simulink model "CaseStudyI_9_Bus"  (R2020a)
settings: Solver=FixedStepAuto  StartTime=0.0  StopTime=Tend  FixedStep=T_s_power  MaxStep=5.0E-5  RelTol=1e-3
values from neighbouring files (symbols this model uses):
  B_s46 = b_s46*Cb    (= 9.5071761847e-07)    [Data_CaseStudyI.m]    (also in Data_CaseStudyII.m; Data_InitialSystem.m)
  B_s54 = b_s54*Cb    (= 1.05902722057e-06)    [Data_CaseStudyI.m]    (also in Data_CaseStudyII.m; Data_InitialSystem.m)
  B_s69 = b_s69*Cb    (= 2.15415764185e-06)    [Data_CaseStudyI.m]    (also in Data_CaseStudyII.m; Data_InitialSystem.m)
  B_s75 = b_s75*Cb    (= 1.84126323577e-06)    [Data_CaseStudyI.m]    (also in Data_CaseStudyII.m; Data_InitialSystem.m)
  B_s87 = b_s87*Cb    (= 8.96562817417e-07)    [Data_CaseStudyI.m]    (also in Data_CaseStudyII.m; Data_InitialSystem.m)
  B_s98 = b_s98*Cb    (= 1.25759482443e-06)    [Data_CaseStudyI.m]    (also in Data_CaseStudyII.m; Data_InitialSystem.m)
  C_dc_DVPP_1_2 = 0.008*(n_DVPP_1_2)    (= 0.8)    [Data_CaseStudyI.m]    (also in Data_CaseStudyII.m)
  C_dc_DVPP_1_3 = 0.008*(n_DVPP_1_3)    (= 0.4)    [Data_CaseStudyI.m]    (also in Data_CaseStudyII.m)
  fb = 50    [Data_CaseStudyI.m]    (also in Data_CaseStudyII.m; Data_InitialSystem.m)
  HGov_dyn = HGov_delay*H_tr_droop    [Data_CaseStudyI.m]    (also in Data_CaseStudyII.m; Data_InitialSystem.m)
  HTurb_tot = H_water_way    [Data_CaseStudyI.m]    (also in Data_CaseStudyII.m; Data_InitialSystem.m)
  I_m_DVPP_1_2 = 2/3*Sb_DVPP_1_2/V_m_DVPP_1_2    [Data_CaseStudyI.m]    (also in Data_CaseStudyII.m)
  I_m_DVPP_1_3 = 2/3*Sb_DVPP_1_3/V_m_DVPP_1_3    [Data_CaseStudyI.m]    (also in Data_CaseStudyII.m)
  i_star_max = 1.3    [Data_CaseStudyI.m]    (also in Data_CaseStudyII.m)
  iabc_DVPP_1_2_0 = T0*idq0_DVPP_1_2    [Data_CaseStudyI.m]    (also in Data_CaseStudyII.m)
  iabc_DVPP_1_3_0 = T0*idq0_DVPP_1_3    [Data_CaseStudyI.m]    (also in Data_CaseStudyII.m)
  K2_DVPP_1 = [-0.0221795494247 -1.60799665656 0.160449825826 -2.94803557381 -11.8081988371 -9.75170960256 0.00463021906909 -49.1667298155]    [ControlGains_DVPP1.mat]
  K3_DVPP_1 = [-0.0591512752956 -1.61493903379 -27.2946107927 -16.2119211358 -14.3657419818 2.05688388773 -2.27328406162 0.146700393037 -150.920793597]    [ControlGains_DVPP1.mat]
  k_dc_DVPP_1_2 = eta_DVPP_1_2/(Vdc_n_DVPP_1_2*m_p_DVPP_1_2)    [Data_CaseStudyI.m]    (also in Data_CaseStudyII.m)
  k_dc_DVPP_1_3 = eta_DVPP_1_3/(Vdc_n_DVPP_1_3*m_p_DVPP_1_3)    [Data_CaseStudyI.m]    (also in Data_CaseStudyII.m)
  ki_i_pu = 1.19    [Data_CaseStudyI.m]    (also in Data_CaseStudyII.m)
  ki_pll = 1700    [Data_CaseStudyI.m]    (also in Data_CaseStudyII.m)
  ki_q_pu = 0.005    [Data_CaseStudyI.m]    (also in Data_CaseStudyII.m)
  kp_i_pu = 0.73    [Data_CaseStudyI.m]    (also in Data_CaseStudyII.m)
  kp_pll = 150    [Data_CaseStudyI.m]    (also in Data_CaseStudyII.m)
  kp_q_pu = 0.05    [Data_CaseStudyI.m]    (also in Data_CaseStudyII.m)
  L1_DVPP_1_2_pu = 0.0186/m_DVPP_1_2    (= 0.000372)    [Data_CaseStudyI.m]    (also in Data_CaseStudyII.m)
  L1_DVPP_1_3_pu = 0.0186/m_DVPP_1_3    (= 0.000744)    [Data_CaseStudyI.m]    (also in Data_CaseStudyII.m)
  l1_MVHV1 = 0    [Data_CaseStudyI.m]    (also in Data_CaseStudyII.m; Data_InitialSystem.m)
  l1_MVHV2 = 0    [Data_CaseStudyI.m]    (also in Data_CaseStudyII.m; Data_InitialSystem.m)
  l1_MVHV3 = 0    [Data_CaseStudyI.m]    (also in Data_CaseStudyII.m; Data_InitialSystem.m)
  L2_DVPP_1_2_pu = L1_DVPP_1_2_pu    (= 0.000372)    [Data_CaseStudyI.m]    (also in Data_CaseStudyII.m)
  L2_DVPP_1_3_pu = L1_DVPP_1_3_pu    (= 0.000744)    [Data_CaseStudyI.m]    (also in Data_CaseStudyII.m)
  l2_MVHV1 = l_s14    (= 0.0576)    [Data_CaseStudyI.m]    (also in Data_CaseStudyII.m; Data_InitialSystem.m)
  l2_MVHV2 = l_s72    (= 0.0625)    [Data_CaseStudyI.m]    (also in Data_CaseStudyII.m; Data_InitialSystem.m)
  l2_MVHV3 = l_s39    (= 0.0586)    [Data_CaseStudyI.m]    (also in Data_CaseStudyII.m; Data_InitialSystem.m)
  l_f_DVPP_1_2 = L_f_DVPP_1_2*w_b/Zb_DVPP_1_2    [Data_CaseStudyI.m]    (also in Data_CaseStudyII.m)
  L_f_DVPP_1_2 = (1/(n_DVPP_1_2))*600*10^-6    (= 6e-06)    [Data_CaseStudyI.m]    (also in Data_CaseStudyII.m)
  l_f_DVPP_1_3 = L_f_DVPP_1_3*w_b/Zb_DVPP_1_3    [Data_CaseStudyI.m]    (also in Data_CaseStudyII.m)
  L_f_DVPP_1_3 = (1/(n_DVPP_1_3))*600*10^-6    (= 1.2e-05)    [Data_CaseStudyI.m]    (also in Data_CaseStudyII.m)
  L_s46 = l_s46*Lb    (= 0.154915055408)    [Data_CaseStudyI.m]    (also in Data_CaseStudyII.m; Data_InitialSystem.m)
  L_s54 = l_s54*Lb    (= 0.143128040323)    [Data_CaseStudyI.m]    (also in Data_CaseStudyII.m; Data_InitialSystem.m)
  L_s69 = l_s69*Lb    (= 0.286256080645)    [Data_CaseStudyI.m]    (also in Data_CaseStudyII.m; Data_InitialSystem.m)
  L_s75 = l_s75*Lb    (= 0.271101346964)    [Data_CaseStudyI.m]    (also in Data_CaseStudyII.m; Data_InitialSystem.m)
  L_s87 = l_s87*Lb    (= 0.12123786945)    [Data_CaseStudyI.m]    (also in Data_CaseStudyII.m; Data_InitialSystem.m)
  L_s98 = l_s98*Lb    (= 0.16973301723)    [Data_CaseStudyI.m]    (also in Data_CaseStudyII.m; Data_InitialSystem.m)
  P_L = pL*Sb    (= 300000000)    [Data_CaseStudyI.m]    (also in Data_CaseStudyII.m; Data_InitialSystem.m)
  p_set_bus1 = P_set_bus1/SbSG1    (= 0.731707317073)    [Data_CaseStudyI.m]    (also in Data_CaseStudyII.m; Data_InitialSystem.m)
  p_set_bus2 = P_set_bus2/SbSG2    (= 0.756707317073)    [Data_CaseStudyI.m]    (also in Data_CaseStudyII.m; Data_InitialSystem.m)
  p_set_bus3 = P_set_bus3/SbSG3    (= 0.731707317073)    [Data_CaseStudyI.m]    (also in Data_CaseStudyII.m; Data_InitialSystem.m)
  pset_DVPP_1_1 = P_set_bus1/SbSG1    (= 0.731707317073)    [Data_CaseStudyI.m]    (also in Data_CaseStudyII.m)
  pset_DVPP_1_2 = 0    [Data_CaseStudyI.m]    (also in Data_CaseStudyII.m)
  pset_DVPP_1_3 = 0    [Data_CaseStudyI.m]    (also in Data_CaseStudyII.m)
  Q_L = qL*Sb    (= 82500000)    [Data_CaseStudyI.m]    (also in Data_CaseStudyII.m; Data_InitialSystem.m)
  qset_DVPP_1_2 = 0    [Data_CaseStudyI.m]    (also in Data_CaseStudyII.m)
  qset_DVPP_1_3 = 0    [Data_CaseStudyI.m]    (also in Data_CaseStudyII.m)
  R1_DVPP_1_2_pu = 0.00734/m_DVPP_1_2    (= 0.0001468)    [Data_CaseStudyI.m]    (also in Data_CaseStudyII.m)
  R1_DVPP_1_3_pu = 0.00734/m_DVPP_1_3    (= 0.0002936)    [Data_CaseStudyI.m]    (also in Data_CaseStudyII.m)
  r1_MVHV1 = 1e-6    (= 1e-06)    [Data_CaseStudyI.m]    (also in Data_CaseStudyII.m; Data_InitialSystem.m)
  r1_MVHV2 = 1e-6    (= 1e-06)    [Data_CaseStudyI.m]    (also in Data_CaseStudyII.m; Data_InitialSystem.m)
  r1_MVHV3 = 1e-6    (= 1e-06)    [Data_CaseStudyI.m]    (also in Data_CaseStudyII.m; Data_InitialSystem.m)
  R2_DVPP_1_2_pu = R1_DVPP_1_2_pu    (= 0.0001468)    [Data_CaseStudyI.m]    (also in Data_CaseStudyII.m)
  R2_DVPP_1_3_pu = R1_DVPP_1_3_pu    (= 0.0002936)    [Data_CaseStudyI.m]    (also in Data_CaseStudyII.m)
  r2_MVHV1 = 1e-6    (= 1e-06)    [Data_CaseStudyI.m]    (also in Data_CaseStudyII.m; Data_InitialSystem.m)
  r2_MVHV2 = 1e-6    (= 1e-06)    [Data_CaseStudyI.m]    (also in Data_CaseStudyII.m; Data_InitialSystem.m)
  r2_MVHV3 = 1e-6    (= 1e-06)    [Data_CaseStudyI.m]    (also in Data_CaseStudyII.m; Data_InitialSystem.m)
  R_dc_DVPP_1_2 = (Vdc_n_DVPP_1_2/(0.05*(Sb_DVPP_1_2)/Vdc_n_DVPP_1_2))    [Data_CaseStudyI.m]    (also in Data_CaseStudyII.m)
  R_dc_DVPP_1_3 = (Vdc_n_DVPP_1_3/(0.05*(Sb_DVPP_1_3)/Vdc_n_DVPP_1_3))    [Data_CaseStudyI.m]    (also in Data_CaseStudyII.m)
  r_f_DVPP_1_2 = R_f_DVPP_1_2/Zb_DVPP_1_2    [Data_CaseStudyI.m]    (also in Data_CaseStudyII.m)
  R_f_DVPP_1_2 = 0.02/n_DVPP_1_2    (= 0.0002)    [Data_CaseStudyI.m]    (also in Data_CaseStudyII.m)
  r_f_DVPP_1_3 = R_f_DVPP_1_3/Zb_DVPP_1_3    [Data_CaseStudyI.m]    (also in Data_CaseStudyII.m)
  R_f_DVPP_1_3 = 0.02/n_DVPP_1_3    (= 0.0004)    [Data_CaseStudyI.m]    (also in Data_CaseStudyII.m)
  R_s46 = r_s46*Zb    (= 8.993)    [Data_CaseStudyI.m]    (also in Data_CaseStudyII.m; Data_InitialSystem.m)
  R_s54 = r_s54*Zb    (= 5.29)    [Data_CaseStudyI.m]    (also in Data_CaseStudyII.m; Data_InitialSystem.m)
  R_s69 = r_s69*Zb    (= 20.631)    [Data_CaseStudyI.m]    (also in Data_CaseStudyII.m; Data_InitialSystem.m)
  R_s75 = r_s75*Zb    (= 16.928)    [Data_CaseStudyI.m]    (also in Data_CaseStudyII.m; Data_InitialSystem.m)
  R_s87 = r_s87*Zb    (= 4.4965)    [Data_CaseStudyI.m]    (also in Data_CaseStudyII.m; Data_InitialSystem.m)
  R_s98 = r_s98*Zb    (= 6.2951)    [Data_CaseStudyI.m]    (also in Data_CaseStudyII.m; Data_InitialSystem.m)
  ReferenceSS2_DVPP_1 = ss(M2T_des_DVPP_1,'minimal')    [Data_CaseStudyI.m]    (also in Data_CaseStudyII.m)
  ReferenceSS3_DVPP_1 = ss(M3T_des_DVPP_1,'minimal')    [Data_CaseStudyI.m]    (also in Data_CaseStudyII.m)
  Rg = 0.03    [Data_CaseStudyI.m]    (also in Data_CaseStudyII.m; Data_InitialSystem.m)
  Sb = 100*10^6    (= 100000000)    [Data_CaseStudyI.m]    (also in Data_CaseStudyII.m; Data_InitialSystem.m)
  Sb_DVPP_1_2 = r_b1*100*10^6*cDVPP_1_2    (= 50000000)    [Data_CaseStudyI.m]    (also in Data_CaseStudyII.m)
  Sb_DVPP_1_3 = r_b1*100*10^6*cDVPP_1_3    (= 25000000)    [Data_CaseStudyI.m]    (also in Data_CaseStudyII.m)
  SbSG1 = r_b1*100*10^6    (= 250000000)    [Data_CaseStudyI.m]    (also in Data_CaseStudyII.m; Data_InitialSystem.m)
  SbSG2 = r_b2*100*10^6    (= 96000000)    [Data_CaseStudyI.m]    (also in Data_CaseStudyII.m; Data_InitialSystem.m)
  SbSG3 = r_b3*100*10^6    (= 64000000)    [Data_CaseStudyI.m]    (also in Data_CaseStudyII.m; Data_InitialSystem.m)
  SGov_dyn = tf([1],[Tg 1])    [Data_CaseStudyI.m]    (also in Data_CaseStudyII.m; Data_InitialSystem.m)
  St_MVHV1 = Sb    (= 100000000)    [Data_CaseStudyI.m]    (also in Data_CaseStudyII.m; Data_InitialSystem.m)
  St_MVHV2 = Sb    (= 100000000)    [Data_CaseStudyI.m]    (also in Data_CaseStudyII.m; Data_InitialSystem.m)
  St_MVHV3 = Sb    (= 100000000)    [Data_CaseStudyI.m]    (also in Data_CaseStudyII.m; Data_InitialSystem.m)
  St_MVLV_DVPP_1_2 = St*m_DVPP_1_2    (= 50000000)    [Data_CaseStudyI.m]    (also in Data_CaseStudyII.m)
  St_MVLV_DVPP_1_3 = St*m_DVPP_1_3    (= 25000000)    [Data_CaseStudyI.m]    (also in Data_CaseStudyII.m)
  STurb_reheat = STurb_ch*STurb_rh    [Data_CaseStudyI.m]    (also in Data_CaseStudyII.m; Data_InitialSystem.m)
  T_load_b3 = 2010    [Data_CaseStudyI.m]    (also in Data_CaseStudyII.m = 1010)
  T_load_b6 = 1010    [Data_CaseStudyI.m]    (also in Data_InitialSystem.m)
  T_s_power = 1e-4    (= 0.0001)    [Data_CaseStudyI.m]    (also in Data_CaseStudyII.m; Data_InitialSystem.m)
  tau_dc_DVPP_1_2 = 0.2    [Data_CaseStudyI.m]    (also in Data_CaseStudyII.m)
  tau_dc_DVPP_1_3 = 0.01    [Data_CaseStudyI.m]    (also in Data_CaseStudyII.m)
  V_m_DVPP_1_2 = VbLV_DVPP_1_2*sqrt(2/3)    [Data_CaseStudyI.m]    (also in Data_CaseStudyII.m)
  V_m_DVPP_1_3 = VbLV_DVPP_1_3*sqrt(2/3)    [Data_CaseStudyI.m]    (also in Data_CaseStudyII.m)
  vabc_DVPP_1_2_0_pu = T0*vdq0_DVPP_1_2_0/V_m_DVPP_1_2    [Data_CaseStudyI.m]    (also in Data_CaseStudyII.m)
  vabc_DVPP_1_3_0_pu = T0*vdq0_DVPP_1_3_0/V_m_DVPP_1_3    [Data_CaseStudyI.m]    (also in Data_CaseStudyII.m)
  VbHV = 230*10^3    (= 230000)    [Data_CaseStudyI.m]    (also in Data_CaseStudyII.m; Data_InitialSystem.m)
  VbLV_DVPP_1_2 = 10^3    (= 1000)    [Data_CaseStudyI.m]    (also in Data_CaseStudyII.m)
  VbLV_DVPP_1_3 = 10^3    (= 1000)    [Data_CaseStudyI.m]    (also in Data_CaseStudyII.m)
  VbMV1 = 16.5*10^3    (= 16500)    [Data_CaseStudyI.m]    (also in Data_CaseStudyII.m; Data_InitialSystem.m)
  VbMV2 = 18.0*10^3    (= 18000)    [Data_CaseStudyI.m]    (also in Data_CaseStudyII.m; Data_InitialSystem.m)
  VbMV3 = 13.8*10^3    (= 13800)    [Data_CaseStudyI.m]    (also in Data_CaseStudyII.m; Data_InitialSystem.m)
  vd0_DVPP_1_2_pu = vd0_DVPP_1_2/V_m_DVPP_1_2    [Data_CaseStudyI.m]    (also in Data_CaseStudyII.m)
  vd0_DVPP_1_3_pu = vd0_DVPP_1_3/V_m_DVPP_1_3    [Data_CaseStudyI.m]    (also in Data_CaseStudyII.m)
  Vdc_n_DVPP_1_2 = 3*V_m_DVPP_1_2    [Data_CaseStudyI.m]    (also in Data_CaseStudyII.m)
  Vdc_n_DVPP_1_3 = 3*V_m_DVPP_1_3    [Data_CaseStudyI.m]    (also in Data_CaseStudyII.m)
  w_b = fb*2*pi    (= 314.159265359)    [Data_CaseStudyI.m]    (also in Data_CaseStudyII.m; Data_InitialSystem.m)
  xid0_DVPP_1_2_pu = 0    [Data_CaseStudyI.m]    (also in Data_CaseStudyII.m)
  xid0_DVPP_1_3_pu = 0    [Data_CaseStudyI.m]    (also in Data_CaseStudyII.m)
  xiq0_DVPP_1_2_pu = 0    [Data_CaseStudyI.m]    (also in Data_CaseStudyII.m)
  xiq0_DVPP_1_3_pu = 0    [Data_CaseStudyI.m]    (also in Data_CaseStudyII.m)
  xpll0_pu = w_b/(ki_pll)    (= 0.184799567858)    [Data_CaseStudyI.m]    (also in Data_CaseStudyII.m)
  xq0_DVPP_1_2_pu = xq0_DVPP_1_2/I_m_DVPP_1_2    [Data_CaseStudyI.m]    (also in Data_CaseStudyII.m)
  ... (+1 more)
undefined symbols (not defined in the file or in its folder): A, B, C, Continuous, Dd, Efd0, gcbh, i_dc, Ka, Kf, p2set, SbSM2, sps_rtmsupport, spsST1AModel, Ta, Tb, Tb1, Tc, Tc1, Tf, VA0, VAmax, VAmin, VImax, VImin, VRmax, VRmin
libraries: powerlib x73, powerlib_meascontrol x16, cstblocks x11, sps_avr x2, simulink_extras x1, simulink x1
(part 2 of 3)

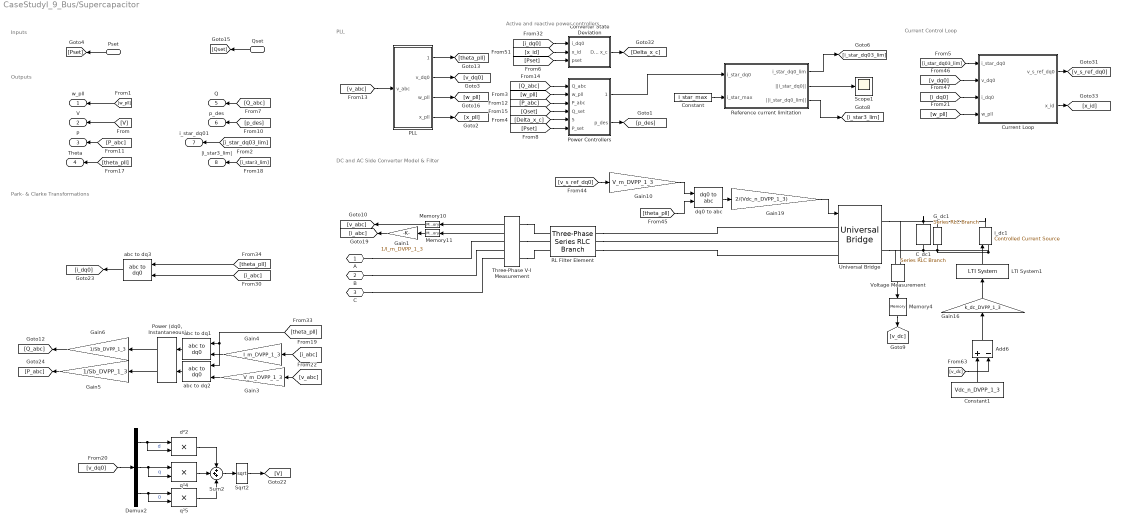
== system CaseStudyI_9_Bus/Supercapacitor ==
  note: Inputs
  note: Active and reactive power controllers
  note: PLL
  note: Outputs
  note: Current Control Loop
  note: Park- & Clarke Transformations
  note: DC and AC Side Converter Model & Filter
  Qset : Inport
  Pset : Inport  Port=2
  Add6 : Sum  Inputs=+-
  C_dc1 : powerlib/Elements/Series RLC Branch  LConnTagsString=__new0  RConnTagsString=__new0  BranchType=C  Resistance=1  Inductance=1e-3  SetiL0=off  InitialCurrent=0  Capacitance=C_dc_DVPP_1_3  Setx0=off  InitialVoltage=Vdc_n  Measurements=None
  Constant : Constant  Value=i_star_max
  Constant1 : Constant  Value=Vdc_n_DVPP_1_3
  Converter State Deviation : Subsystem
  Current Loop : Subsystem  AncestorBlock=Library/Grid-Forming Converter Controlled by Droop Control /Current Loop
  Demux2 : Demux  Outputs=3
  G_dc1 : powerlib/Elements/Series RLC Branch  LConnTagsString=__new0  RConnTagsString=__new0  BranchType=R  Resistance=R_dc_DVPP_1_3  Inductance=1e-3  SetiL0=off  InitialCurrent=0  Capacitance=1e-6  Setx0=off  InitialVoltage=0  Measurements=None
  Gain1 : Gain  Gain=1/I_m_DVPP_1_3
  Gain10 : Gain  Gain=V_m_DVPP_1_3
  Gain16 : Gain  Gain=k_dc_DVPP_1_3
  Gain19 : Gain  Gain=2/(Vdc_n_DVPP_1_3)
  Gain3 : Gain  Gain=V_m_DVPP_1_3
  Gain4 : Gain  Gain=I_m_DVPP_1_3
  Gain5 : Gain  Gain=1/Sb_DVPP_1_3
  Gain6 : Gain  Gain=1/Sb_DVPP_1_3
  LTI System1 : cstblocks/LTI System  sys=tf(1,[tau_dc_DVPP_1_3 1])  IC=[]
  Memory10 : Memory  InitialCondition=[vabc_DVPP_1_3_0_pu(1), vabc_DVPP_1_3_0_pu(2), vabc_DVPP_1_3_0_pu(3)]
  Memory11 : Memory  InitialCondition=[iabc_DVPP_1_3_0(1), iabc_DVPP_1_3_0(2), iabc_DVPP_1_3_0(3)]
  Memory4 : Memory
  PLL : Subsystem
  "Power (dq0, Instantaneous)" : powerlib_meascontrol/Measurements/Power (dq0, Instantaneous)
      settings: SourceProductBaseCode=PS
  Power Controllers : Subsystem
  RL Filter Element : powerlib/Elements/Three-Phase Series RLC Branch  LConnTagsString=A|B|C  RConnTagsString=A|B|C  BranchType=RL  Resistance=R_f_DVPP_1_3  Inductance=L_f_DVPP_1_3  Capacitance=0  Measurements=Branch currents
  Reference current limitation : Subsystem
  Scope1 : Scope
  Sqrt2 : Sqrt  SaturateOnIntegerOverflow=on
  Sum2 : Sum  Inputs=+++  InputSameDT=on  SaturateOnIntegerOverflow=on  OutDataTypeStr=Inherit: Same as first input
  Three-Phase V-I Measurement : powerlib/Measurements/Three-Phase V-I Measurement  VoltageMeasurement=phase-to-ground  SetLabelV=off  LabelV=Vabc  Vpu=on  VpuLL=off  CurrentMeasurement=yes  SetLabelI=off  LabelI=Iabc  Ipu=off  Pbase=Sb_conv  Vbase=VbLV_DVPP_1_3  OutputType=Complex  PhasorSimulation=off  PSBequivalent=0
  Universal Bridge : powerlib/Power Electronics/Universal Bridge  Arms=3  SnubberResistance=1e5  SnubberCapacitance=inf  Device=Average-model based VSC  Ron=1e-3  Lon=0  ForwardVoltages="[  0  0  ]"  ForwardVoltage=0  GTOparameters=[ 10e-6 , 20e-6 ]  IGBTparameters=[ 1e-6 , 2e-6 ]  Measurements=None  Measurements_2=None  converterType=Rectifier
  Voltage Measurement : powerlib/Measurements/Voltage Measurement  PhasorSimulation=off  OutputType=Complex  PSBequivalent=0
  abc to dq1 : powerlib_meascontrol/Transformations/abc to dq0  Alignment=90 degrees behind phase A axis
  abc to dq2 : powerlib_meascontrol/Transformations/abc to dq0  Alignment=90 degrees behind phase A axis
  abc to dq3 : powerlib_meascontrol/Transformations/abc to dq0  Alignment=90 degrees behind phase A axis
  dq0 to abc : powerlib_meascontrol/Transformations/dq0 to abc  Alignment=90 degrees behind phase A axis
  d²2 : Product  InputSameDT=on  RndMeth=Zero  SaturateOnIntegerOverflow=on  OutDataTypeStr=Inherit: Same as first input
  i_dc1 : powerlib/Electrical Sources/Controlled Current Source  Initialize=off  Source_Type=DC  Amplitude=i_dc  Phase=0  Frequency=0  Measurements=None
  q²4 : Product  InputSameDT=on  RndMeth=Zero  SaturateOnIntegerOverflow=on  OutDataTypeStr=Inherit: Same as first input
  q²5 : Product  InputSameDT=on  RndMeth=Zero  SaturateOnIntegerOverflow=on  OutDataTypeStr=Inherit: Same as first input
  A : PMIOPort  Side=Right
  B : PMIOPort  Port=2  Side=Right
  C : PMIOPort  Port=3  Side=Right
  w_pll : Outport  VectorParamsAs1DForOutWhenUnconnected=off
  V : Outport  Port=2  VectorParamsAs1DForOutWhenUnconnected=off
  P : Outport  Port=3  VectorParamsAs1DForOutWhenUnconnected=off
  Theta : Outport  Port=4  VectorParamsAs1DForOutWhenUnconnected=off
  Q : Outport  Port=5  VectorParamsAs1DForOutWhenUnconnected=off
  p_des : Outport  Port=6  VectorParamsAs1DForOutWhenUnconnected=off
  i_star_dq01 : Outport  Port=7  VectorParamsAs1DForOutWhenUnconnected=off
  |i_star3_lim| : Outport  Port=8  VectorParamsAs1DForOutWhenUnconnected=off
  wires:
  PLL/4(x_pll) -> [x_pll]
  [v_abc] -> PLL/1(v_abc)
  [i_star_dq03_lim] -> i_star_dq01/1
  PLL/2(v_dq0) -> [v_dq0]
  [p_des] -> p_des/1
  PLL/1(theta_pll) -> [theta_pll]
  PLL/3(w_pll) -> [w_pll]
  [V] -> V/1
  [w_pll] -> w_pll/1
  [theta_pll] -> Theta/1
  Power Controllers/2(p_des) -> [p_des]
  [Q_abc] -> Q/1
  Qset/1 -> [Qset]
  [P_abc] -> P/1
  Constant/1 -> Reference current limitation/2(i_star_max)
  Reference current limitation/2(||i_star_dq0||) -> Scope1/1
  [i_star3_lim] -> |i_star3_lim|/1
  [w_pll] -> Current Loop/4(w_pll)
  [i_dq0] -> Current Loop/3(i_dq0)
  Reference current limitation/1(i_star_dq0_lim) -> [i_star_dq03_lim]
  [v_dq0] -> Current Loop/2(v_dq0)
  [v_dq0] -> Demux2/1
  Sum2/1 -> Sqrt2/1
  [i_abc] -> Gain4/1
  Demux2/3 -> q²5/2, q²5/1  "0"
  Gain1/1 -> [i_abc]
  Memory11/1 -> Gain1/1
  Demux2/1 -> d²2/1, d²2/2  "d"
  Three-Phase V-I Measurement/2 -> Memory11/1
  abc to dq1/1 -> "Power (dq0, Instantaneous)"/2
  Three-Phase V-I Measurement/1 -> Memory10/1
  Gain5/1 -> [P_abc]
  Gain4/1 -> abc to dq1/1
  Gain3/1 -> abc to dq2/1
  q²4/1 -> Sum2/2
  Gain6/1 -> [Q_abc]
  Gain19/1 -> Universal Bridge/1
  Add6/1 -> Gain16/1
  LTI System1/1 -> i_dc1/1
  [v_abc] -> Gain3/1
  [theta_pll] -> abc to dq3/2
  abc to dq3/1 -> [i_dq0]
  Voltage Measurement/1 -> Memory4/1
  d²2/1 -> Sum2/1
  [theta_pll] -> abc to dq2/2, abc to dq1/2
  dq0 to abc/1 -> Gain19/1
  Memory10/1 -> [v_abc]
  "Power (dq0, Instantaneous)"/2 -> Gain6/1
  Sqrt2/1 -> [V]
  "Power (dq0, Instantaneous)"/1 -> Gain5/1
  Demux2/2 -> q²4/1, q²4/2  "q"
  [v_dc] -> Add6/2
  q²5/1 -> Sum2/3
  abc to dq2/1 -> "Power (dq0, Instantaneous)"/1
  Memory4/1 -> [v_dc]
  Gain10/1 -> dq0 to abc/1
  [theta_pll] -> dq0 to abc/2
  [i_abc] -> abc to dq3/1
  [v_s_ref_dq0] -> Gain10/1
  Gain16/1 -> LTI System1/1
  Constant1/1 -> Add6/1
  Current Loop/2(x_id) -> [x_id]
  Current Loop/1(v_s_ref_dq0) -> [v_s_ref_dq0]
  [P_abc] -> Power Controllers/3(P_abc)
  [w_pll] -> Power Controllers/2(w_pll)
  [Delta_x_c] -> Power Controllers/5(Delta x_c)
  [Q_abc] -> Power Controllers/1(Q_abc)
  [Qset] -> Power Controllers/4(Q_set)
  Reference current limitation/3(||i_star_dq0_lim||) -> [i_star3_lim]
  [i_star_dq03_lim] -> Current Loop/1(i_star_dq0)
  Power Controllers/1(i_star_dq0) -> Reference current limitation/1(i_star_dq0)
  [Pset] -> Converter State Deviation/3(pset)
  [x_id] -> Converter State Deviation/2(x_id)
  [i_dq0] -> Converter State Deviation/1(i_dq0)
  Converter State Deviation/1(Delta x_c) -> [Delta_x_c]
  [Pset] -> Power Controllers/6(P_set)
  Pset/1 -> [Pset]
  connections:
  i_dc1/LConn1 -- G_dc1/RConn1 -- Voltage Measurement/LConn2 -- Universal Bridge/RConn2 -- C_dc1/RConn1
  i_dc1/RConn1 -- Universal Bridge/RConn1 -- Voltage Measurement/LConn1 -- C_dc1/LConn1 -- G_dc1/LConn1
  Three-Phase V-I Measurement/LConn2 -- RL Filter Element/LConn2
  RL Filter Element/RConn3 -- Universal Bridge/LConn3
  B/RConn1 -- Three-Phase V-I Measurement/RConn2
  C/RConn1 -- Three-Phase V-I Measurement/RConn3
  Three-Phase V-I Measurement/LConn1 -- RL Filter Element/LConn1
  RL Filter Element/RConn2 -- Universal Bridge/LConn2
  A/RConn1 -- Three-Phase V-I Measurement/RConn1
  Three-Phase V-I Measurement/LConn3 -- RL Filter Element/LConn3
  RL Filter Element/RConn1 -- Universal Bridge/LConn1

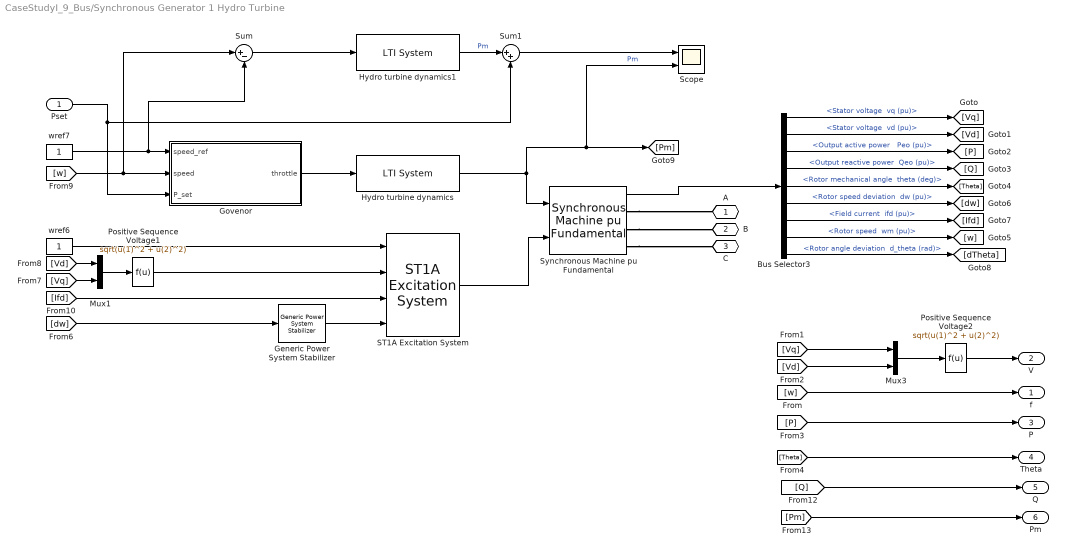
== system CaseStudyI_9_Bus/Synchronous Generator 1 Hydro Turbine ==
  Pset : Inport
  Bus Selector3 : BusSelector  OutputSignals="dq0 components.Stator voltage  vq (pu),dq0 components.Stator voltage  vd (pu),Output active power   Peo (pu),Output reactive power  Qeo (pu),Mechanical.Rotor mechanical angle  theta (deg),Mechanical.Rotor speed deviation  dw (pu),dq0 components.Field current  ifd (pu),Mechanical.Rotor speed  wm (pu),Mechanical.Rotor angle deviation  d_theta (rad)"
  Generic Power System Stabilizer : powerlib/Machines/Generic Power System Stabilizer  Tsensor=30e-3  K=15  Twashout=1  Tleadlag1=[50e-3 20e-3]  Tleadlag2=[3 5.4]  VSlimits=[-0.15 0.15]  Vinit=0  Plot_On=off  MagdB_On=on  FreqRange=logspace(-2,2,500)
      settings: SourceProductBaseCode=PS
  Govenor : Subsystem
  Hydro turbine dynamics : cstblocks/LTI System  sys=ss(HTurb_tot)  IC=p_set_bus1/3
  Hydro turbine dynamics1 : cstblocks/LTI System  sys=M1T_des_DVPP_1  IC=p_set_bus1/3
  Mux1 : Mux  Inputs=2
  Mux3 : Mux  Inputs=2
  Positive Sequence Voltage1 : Fcn  Expr=sqrt(u(1)^2 + u(2)^2)
  Positive Sequence Voltage2 : Fcn  Expr=sqrt(u(1)^2 + u(2)^2)
  ST1A Excitation System : sps_avr/ST1A Excitation System  Tr=20e-3  KaTa=[210 0.001]  VIminmax=[-999 +999]  VAminmax=[-999 999]  VRminmax=[-6.0 6.43]  KfTf=[0.001 1]  TbTc=[0 0 0 0]  KLR=1  ILR=2  Kc=0.038  v0=[1 1.7165]  TsBlock=0
      settings: SourceProductBaseCode=PS
  Scope : Scope  NumInputPorts=2
  Sum : Sum  Inputs=|+-
  Sum1 : Sum  Inputs=|++
  Synchronous Machine pu Fundamental : powerlib/Machines/Synchronous Machine pu Fundamental  PresetModel=No  MechanicalLoad=Mechanical power Pm  ShowDetailedParameters=on  RotorType=Round  Units=per unit fundamental parameters  MeasurementBus=off  NominalParameters="[SbSG1  VbMV1   fb]"  Stator="[ 2.85E-03  0.114  1.19  0.36 ]"  Field="[ 5.79E-04  0.114]"  Dampers2=[0.0652, 0.5134, 0.0287, 0.2553, 7.765e-3, 0.9167 ]  Dampers1="[ 1.17E-02  0.182  1.97E-02  0.384 ]"  Mechanical=[6 0.0032 20]  PolePairs=20  InitialConditions=[0 0 0 0 0 0 0 0 1]  SetSaturation=off  Saturation=[0.6404,0.7127,0.8441,0.9214,0.9956,1.082,1.19,1.316,1.457;0.7,0.7698,0.8872,0.9466,0.9969,1.046,1.1,1.151,1.201]  LoadFlowParameters=[1,0,0,0,0]  TsPowergui=0  TsBlock=-1  IterativeModel=Trapezoidal non iterative  IterativeDiscreteModel=Trapezoidal non iterative  BusType=swing  Pref=p2set*SbSM2  Qref=0  Qmin=-inf  Qmax=inf  PLF=0  QLF=0
      settings: SourceProductBaseCode=PS
  wref6 : Constant
  wref7 : Constant
  A : PMIOPort  Side=Right
  B : PMIOPort  Port=2  Side=Right
  C : PMIOPort  Port=3  Side=Right
  f : Outport  VectorParamsAs1DForOutWhenUnconnected=off
  V : Outport  Port=2  VectorParamsAs1DForOutWhenUnconnected=off
  P : Outport  Port=3  VectorParamsAs1DForOutWhenUnconnected=off
  Theta : Outport  Port=4  VectorParamsAs1DForOutWhenUnconnected=off
  Q : Outport  Port=5  VectorParamsAs1DForOutWhenUnconnected=off
  Pm : Outport  Port=6  VectorParamsAs1DForOutWhenUnconnected=off
  wires:
  ST1A Excitation System/1 -> Synchronous Machine pu Fundamental/2
  [dw] -> Generic Power System Stabilizer/1
  Bus Selector3/8 -> [w]  "<Rotor speed  wm (pu)>"
  Bus Selector3/7 -> [Ifd]  "<Field current  ifd (pu)>"
  Bus Selector3/6 -> [dw]  "<Rotor speed deviation  dw (pu)>"
  Bus Selector3/5 -> [Theta]  "<Rotor mechanical angle  theta (deg)>"
  Bus Selector3/4 -> [Q]  "<Output reactive power  Qeo (pu)>"
  Bus Selector3/3 -> [P]  "<Output active power   Peo (pu)>"
  Bus Selector3/2 -> [Vd]  "<Stator voltage  vd (pu)>"
  Bus Selector3/1 -> [Vq]  "<Stator voltage  vq (pu)>"
  [Theta] -> Theta/1
  [P] -> P/1
  [Vd] -> Mux3/2
  [Vq] -> Mux3/1
  Synchronous Machine pu Fundamental/1 -> Bus Selector3/1
  Mux3/1 -> Positive Sequence Voltage2/1
  wref6/1 -> ST1A Excitation System/1
  Positive Sequence Voltage2/1 -> V/1
  [w] -> f/1
  Bus Selector3/9 -> [dTheta]  "<Rotor angle deviation  d_theta (rad)>"
  Mux1/1 -> Positive Sequence Voltage1/1
  [Vd] -> Mux1/1
  [Vq] -> Mux1/2
  Generic Power System Stabilizer/1 -> ST1A Excitation System/4
  Govenor/1(throttle) -> Hydro turbine dynamics/1
  [Q] -> Q/1
  Positive Sequence Voltage1/1 -> ST1A Excitation System/2
  [Ifd] -> ST1A Excitation System/3
  wref7/1 -> Sum/2, Govenor/1(speed_ref)
  Pset/1 -> Sum1/2, Govenor/3(P_set)
  [Pm] -> Pm/1
  [w] -> Sum/1, Govenor/2(speed)
  Hydro turbine dynamics/1 -> Synchronous Machine pu Fundamental/1, Scope/2, [Pm]  "Pm"
  Sum/1 -> Hydro turbine dynamics1/1
  Hydro turbine dynamics1/1 -> Sum1/1  "Pm"
  Sum1/1 -> Scope/1
  connections:
  Synchronous Machine pu Fundamental/RConn2 -- B/RConn1
  Synchronous Machine pu Fundamental/RConn3 -- C/RConn1
  Synchronous Machine pu Fundamental/RConn1 -- A/RConn1

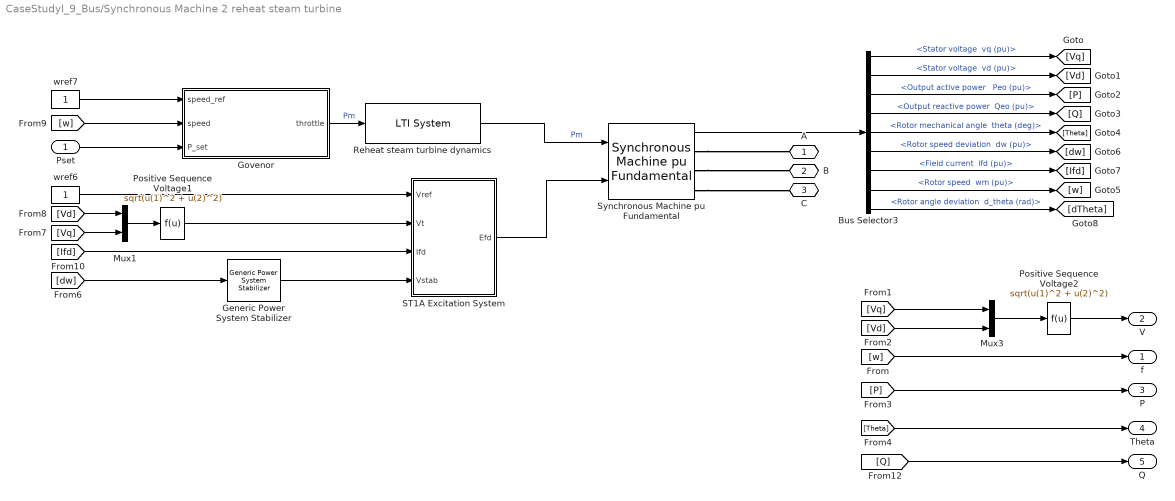
== system CaseStudyI_9_Bus/Synchronous Machine 2 reheat steam turbine ==
  Pset : Inport
  Bus Selector3 : BusSelector  OutputSignals="dq0 components.Stator voltage  vq (pu),dq0 components.Stator voltage  vd (pu),Output active power   Peo (pu),Output reactive power  Qeo (pu),Mechanical.Rotor mechanical angle  theta (deg),Mechanical.Rotor speed deviation  dw (pu),dq0 components.Field current  ifd (pu),Mechanical.Rotor speed  wm (pu),Mechanical.Rotor angle deviation  d_theta (rad)"
  Generic Power System Stabilizer : powerlib/Machines/Generic Power System Stabilizer  Tsensor=30e-3  K=15  Twashout=1  Tleadlag1=[50e-3 20e-3]  Tleadlag2=[3 5.4]  VSlimits=[-0.15 0.15]  Vinit=0  Plot_On=off  MagdB_On=on  FreqRange=logspace(-2,2,500)
      settings: SourceProductBaseCode=PS
  Govenor : Subsystem
  Mux1 : Mux  Inputs=2
  Mux3 : Mux  Inputs=2
  Positive Sequence Voltage1 : Fcn  Expr=sqrt(u(1)^2 + u(2)^2)
  Positive Sequence Voltage2 : Fcn  Expr=sqrt(u(1)^2 + u(2)^2)
  Reheat steam turbine dynamics : cstblocks/LTI System  sys=ss(STurb_reheat)  IC=[1 0.2281]
  ST1A Excitation System : Subsystem  AncestorBlock=sps_avr/ST1A Excitation System  DialogController=POWERSYS.PowerSysDialog  LoadFcn=sps_rtmsupport('LoadFcn', gcbh);  StartFcn=sps_rtmsupport('StartFcn', gcbh);  StopFcn=sps_rtmsupport('StopFcn', gcbh);  mask(ST1A Excitation System){Tr=20e-3, KaTa=[210 0.001], VIminmax=[-999 +999], VAminmax=[-999 999], VRminmax=[-6.0 6.43], KfTf=[0.001 1], TbTc=[0 0 0 0], KLR=1, ILR=2, Kc=0.038, v0=[1 1.6825], TsBlock=0}
      mask prompts: Tr "Low-pass filter time constant Tr(s):"; KaTa "Voltage regulator gain and time constant [Ka Ta(s)]:"; VIminmax "Voltage regulator input limits [VImin(pu) VImax(pu)]:"; VAminmax "Voltage regulator internal limits [VAmin(pu) VAmax(pu)]:"; VRminmax "Voltage regulator output limits [VRmin(pu) VRmax(pu)]:"; KfTf "Damping filter gain and time constant [Kf Tf(s)]:"; TbTc "Transient gain reduction lead and lag time constants [Tb(s) Tc(s) Tb1(s) Tc1(s)]:"; KLR "Exciter output current limiter gain KLR(pu):"; ILR "Exciter output current limit reference ILR(pu):"; Kc "Rectifier loading factor Kc(pu):"; v0 "Initial values of terminal voltage and field voltage [Vt0(pu) Efd0(pu)]:"; TsBlock "Sample time:"
      mask help: Implements a synchronous machine voltage regulator and exciter based on the IEEE type ST1A excitation system model. The output is the field voltage to apply to the Vf input of a Synchronous Machine block. Inputs and output are in p.u.
      mask init:
      | block = gcb;
      | [Ts,BlockChoice,MaskType,Ka,Ta,Kf,Tf,Tb,Tc,Tb1,Tc1,VRmin,VRmax,VImin,VImax,VAmin,VAmax,Ifd0,VA0,Vt0,Efd0] = powericon('ExcitationSystemInit',block,TsBlock,KaTa,KfTf,TbTc,VRminmax,VIminmax,VAminmax,Kc,ILR,KLR,v0);
      | powericon('SetInternalModels','set',block,BlockChoice);
      settings: CopyFcn=sps_rtmsupport('CopyFcn', gcbh);  DeleteFcn=sps_rtmsupport('DeleteFcn', gcbh);  UndoDeleteFcn=sps_rtmsupport('UndoDeleteFcn', gcbh);  ModelCloseFcn=sps_rtmsupport('ModelCloseFcn', gcbh);  PreSaveFcn=sps_rtmsupport('PreSaveFcn', gcbh);  PostSaveFcn=sps_rtmsupport('PostSaveFcn', gcbh);  NameChangeFcn=sps_rtmsupport('NameChangeFcn', gcbh);  PreCopyFcn=sps_rtmsupport('PreCopyFcn', gcbh);  OpenFcn=sps_rtmsupport('OpenFcn', gcbh, []);  CloseFcn=sps_rtmsupport('CloseFcn', gcbh);  PreDeleteFcn=sps_rtmsupport('PreDeleteFcn', gcbh);
      mask Help: helpview(psbhelp);
      mask Display: color('blue');disp('ST1A')
  Synchronous Machine pu Fundamental : powerlib/Machines/Synchronous Machine pu Fundamental  PresetModel=No  MechanicalLoad=Mechanical power Pm  ShowDetailedParameters=on  RotorType=Round  Units=per unit fundamental parameters  MeasurementBus=off  NominalParameters="[ SbSG2  VbMV2   fb]"  Stator="[ 2.85E-03  0.114  1.19  0.36 ]"  Field="[ 5.79E-04  0.114]"  Dampers2=[0.0652, 0.5134, 0.0287, 0.2553, 7.765e-3, 0.9167 ]  Dampers1="[ 1.17E-02  0.182  1.97E-02  0.384 ]"  Mechanical=[13 0 20]  PolePairs=20  InitialConditions=[0 0 0 0 0 0 0 0 1]  SetSaturation=off  Saturation=[0.6404,0.7127,0.8441,0.9214,0.9956,1.082,1.19,1.316,1.457;0.7,0.7698,0.8872,0.9466,0.9969,1.046,1.1,1.151,1.201]  LoadFlowParameters=[1,0,0,0,0]  TsPowergui=0  TsBlock=-1  IterativeModel=Trapezoidal non iterative  IterativeDiscreteModel=Trapezoidal non iterative  BusType=PV  Pref=P_set_bus2  Qref=0  Qmin=-inf  Qmax=inf  PLF=0  QLF=0
      settings: SourceProductBaseCode=PS
  wref6 : Constant
  wref7 : Constant
  A : PMIOPort  Side=Right
  B : PMIOPort  Port=2  Side=Right
  C : PMIOPort  Port=3  Side=Right
  f : Outport  VectorParamsAs1DForOutWhenUnconnected=off
  V : Outport  Port=2  VectorParamsAs1DForOutWhenUnconnected=off
  P : Outport  Port=3  VectorParamsAs1DForOutWhenUnconnected=off
  Theta : Outport  Port=4  VectorParamsAs1DForOutWhenUnconnected=off
  Q : Outport  Port=5  VectorParamsAs1DForOutWhenUnconnected=off
  wires:
  ST1A Excitation System/1(Efd) -> Synchronous Machine pu Fundamental/2
  [dw] -> Generic Power System Stabilizer/1
  Generic Power System Stabilizer/1 -> ST1A Excitation System/4(Vstab)
  Bus Selector3/8 -> [w]  "<Rotor speed  wm (pu)>"
  Bus Selector3/7 -> [Ifd]  "<Field current  ifd (pu)>"
  Bus Selector3/6 -> [dw]  "<Rotor speed deviation  dw (pu)>"
  Bus Selector3/5 -> [Theta]  "<Rotor mechanical angle  theta (deg)>"
  Bus Selector3/4 -> [Q]  "<Output reactive power  Qeo (pu)>"
  Bus Selector3/3 -> [P]  "<Output active power   Peo (pu)>"
  Bus Selector3/2 -> [Vd]  "<Stator voltage  vd (pu)>"
  Bus Selector3/1 -> [Vq]  "<Stator voltage  vq (pu)>"
  [Theta] -> Theta/1
  [P] -> P/1
  [Vd] -> Mux3/2
  [Vq] -> Mux3/1
  Synchronous Machine pu Fundamental/1 -> Bus Selector3/1
  Mux3/1 -> Positive Sequence Voltage2/1
  wref6/1 -> ST1A Excitation System/1(Vref)
  Positive Sequence Voltage2/1 -> V/1
  [w] -> f/1
  Bus Selector3/9 -> [dTheta]  "<Rotor angle deviation  d_theta (rad)>"
  Mux1/1 -> Positive Sequence Voltage1/1
  [Vd] -> Mux1/1
  [Vq] -> Mux1/2
  [w] -> Govenor/2(speed)
  wref7/1 -> Govenor/1(speed_ref)
  [Q] -> Q/1
  Govenor/1(throttle) -> Reheat steam turbine dynamics/1  "Pm"
  Positive Sequence Voltage1/1 -> ST1A Excitation System/2(Vt)
  [Ifd] -> ST1A Excitation System/3(Ifd)
  Pset/1 -> Govenor/3(P_set)
  Reheat steam turbine dynamics/1 -> Synchronous Machine pu Fundamental/1  "Pm"
  connections:
  Synchronous Machine pu Fundamental/RConn2 -- B/RConn1
  Synchronous Machine pu Fundamental/RConn3 -- C/RConn1
  Synchronous Machine pu Fundamental/RConn1 -- A/RConn1

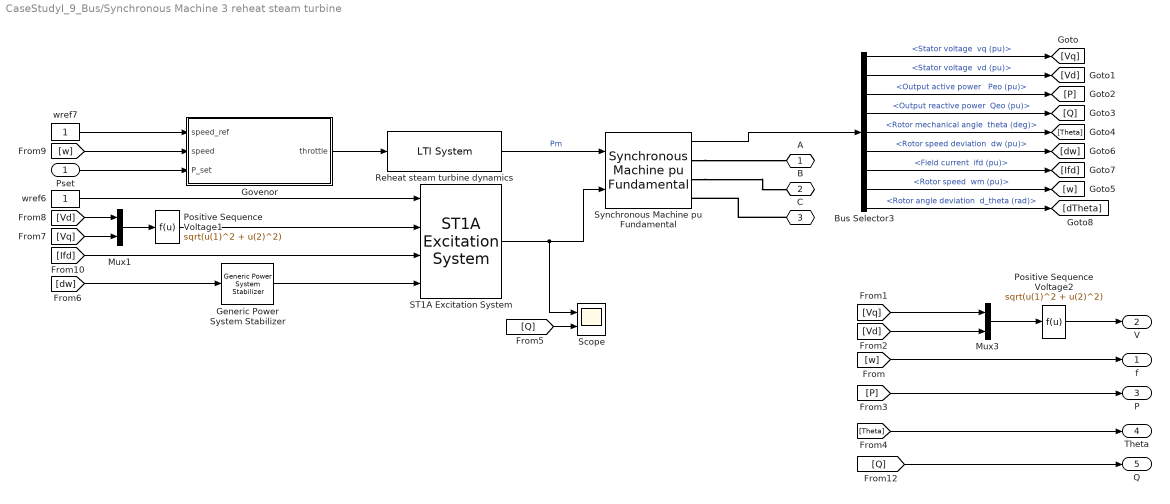
== system CaseStudyI_9_Bus/Synchronous Machine 3 reheat steam turbine ==
  Pset : Inport
  Bus Selector3 : BusSelector  OutputSignals="dq0 components.Stator voltage  vq (pu),dq0 components.Stator voltage  vd (pu),Output active power   Peo (pu),Output reactive power  Qeo (pu),Mechanical.Rotor mechanical angle  theta (deg),Mechanical.Rotor speed deviation  dw (pu),dq0 components.Field current  ifd (pu),Mechanical.Rotor speed  wm (pu),Mechanical.Rotor angle deviation  d_theta (rad)"
  Generic Power System Stabilizer : powerlib/Machines/Generic Power System Stabilizer  Tsensor=30e-3  K=15  Twashout=1  Tleadlag1=[50e-3 20e-3]  Tleadlag2=[3 5.4]  VSlimits=[-0.15 0.15]  Vinit=0  Plot_On=off  MagdB_On=on  FreqRange=logspace(-2,2,500)
      settings: SourceProductBaseCode=PS
  Govenor : Subsystem
  Mux1 : Mux  Inputs=2
  Mux3 : Mux  Inputs=2
  Positive Sequence Voltage1 : Fcn  Expr=sqrt(u(1)^2 + u(2)^2)
  Positive Sequence Voltage2 : Fcn  Expr=sqrt(u(1)^2 + u(2)^2)
  Reheat steam turbine dynamics : cstblocks/LTI System  sys=ss(STurb_reheat)  IC=[1 0.2281]
  ST1A Excitation System : sps_avr/ST1A Excitation System  Tr=20e-3  KaTa=[210 0.001]  VIminmax=[-999 +999]  VAminmax=[-999 999]  VRminmax=[-6.0 6.43]  KfTf=[0.001 1]  TbTc=[0 0 0 0]  KLR=1  ILR=2  Kc=0.038  v0=[1 1.64]  TsBlock=0
      settings: SourceProductBaseCode=PS
  Scope : Scope  NumInputPorts=2
  Synchronous Machine pu Fundamental : powerlib/Machines/Synchronous Machine pu Fundamental  PresetModel=No  MechanicalLoad=Mechanical power Pm  ShowDetailedParameters=on  RotorType=Round  Units=per unit fundamental parameters  MeasurementBus=off  NominalParameters="[ SbSG3 VbMV3   fb]"  Stator="[ 2.85E-03  0.114  1.19  0.36 ]"  Field="[ 5.79E-04  0.114]"  Dampers2=[0.0652, 0.5134, 0.0287, 0.2553, 7.765e-3, 0.9167 ]  Dampers1="[ 1.17E-02  0.182  1.97E-02  0.384 ]"  Mechanical=[13 0 20]  PolePairs=20  InitialConditions=[0 -61.0946 1.01786 1.01786 1.01786 6.04511 -113.955 126.045 1.41461]  SetSaturation=off  Saturation=[0.6404,0.7127,0.8441,0.9214,0.9956,1.082,1.19,1.316,1.457;0.7,0.7698,0.8872,0.9466,0.9969,1.046,1.1,1.151,1.201]  LoadFlowParameters=[1,0,0,0,0]  TsPowergui=0  TsBlock=-1  IterativeModel=Trapezoidal non iterative  IterativeDiscreteModel=Trapezoidal non iterative  BusType=PV  Pref=P_set_bus3  Qref=0  Qmin=-inf  Qmax=inf  PLF=0  QLF=0
      settings: SourceProductBaseCode=PS
  wref6 : Constant
  wref7 : Constant
  A : PMIOPort  Side=Right
  B : PMIOPort  Port=2  Side=Right
  C : PMIOPort  Port=3  Side=Right
  f : Outport  VectorParamsAs1DForOutWhenUnconnected=off
  V : Outport  Port=2  VectorParamsAs1DForOutWhenUnconnected=off
  P : Outport  Port=3  VectorParamsAs1DForOutWhenUnconnected=off
  Theta : Outport  Port=4  VectorParamsAs1DForOutWhenUnconnected=off
  Q : Outport  Port=5  VectorParamsAs1DForOutWhenUnconnected=off
  wires:
  ST1A Excitation System/1 -> Scope/1, Synchronous Machine pu Fundamental/2
  [dw] -> Generic Power System Stabilizer/1
  Generic Power System Stabilizer/1 -> ST1A Excitation System/4
  Bus Selector3/8 -> [w]  "<Rotor speed  wm (pu)>"
  Bus Selector3/7 -> [Ifd]  "<Field current  ifd (pu)>"
  Bus Selector3/6 -> [dw]  "<Rotor speed deviation  dw (pu)>"
  Bus Selector3/5 -> [Theta]  "<Rotor mechanical angle  theta (deg)>"
  Bus Selector3/4 -> [Q]  "<Output reactive power  Qeo (pu)>"
  Bus Selector3/3 -> [P]  "<Output active power   Peo (pu)>"
  Bus Selector3/2 -> [Vd]  "<Stator voltage  vd (pu)>"
  Bus Selector3/1 -> [Vq]  "<Stator voltage  vq (pu)>"
  [Theta] -> Theta/1
  [P] -> P/1
  [Vd] -> Mux3/2
  [Vq] -> Mux3/1
  Synchronous Machine pu Fundamental/1 -> Bus Selector3/1
  Mux3/1 -> Positive Sequence Voltage2/1
  wref6/1 -> ST1A Excitation System/1
  Positive Sequence Voltage2/1 -> V/1
  [w] -> f/1
  Bus Selector3/9 -> [dTheta]  "<Rotor angle deviation  d_theta (rad)>"
  Mux1/1 -> Positive Sequence Voltage1/1
  [Vq] -> Mux1/2
  [Vd] -> Mux1/1
  Govenor/1(throttle) -> Reheat steam turbine dynamics/1
  [w] -> Govenor/2(speed)
  Reheat steam turbine dynamics/1 -> Synchronous Machine pu Fundamental/1  "Pm"
  wref7/1 -> Govenor/1(speed_ref)
  [Q] -> Q/1
  Pset/1 -> Govenor/3(P_set)
  [Q] -> Scope/2
  [Ifd] -> ST1A Excitation System/3
  Positive Sequence Voltage1/1 -> ST1A Excitation System/2
  connections:
  Synchronous Machine pu Fundamental/RConn2 -- B/RConn1
  C/RConn1 -- Synchronous Machine pu Fundamental/RConn3
  Synchronous Machine pu Fundamental/RConn1 -- A/RConn1

== system CaseStudyI_9_Bus/BESS/Converter State Deviation ==
  i_dq0 : Inport
  x_id : Inport  Port=2
  pset : Inport  Port=3
  Constant1 : Constant  Value=xid0_DVPP_1_2_pu
  Demux2 : Demux  Outputs=3
  Gain : Gain  Gain=1/vd0_DVPP_1_2_pu
  Mux : Mux  Inputs=2
  Sum : Sum  Inputs=-+|
  Sum1 : Sum  Inputs=|+-
  Delta x_c : Outport
  wires:
  i_dq0/1 -> Demux2/1
  pset/1 -> Gain/1
  Sum/1 -> Mux/1
  Demux2/1 -> Sum/2
  Gain/1 -> Sum/1
  x_id/1 -> Sum1/1
  Constant1/1 -> Sum1/2
  Mux/1 -> Delta x_c/1
  Sum1/1 -> Mux/2

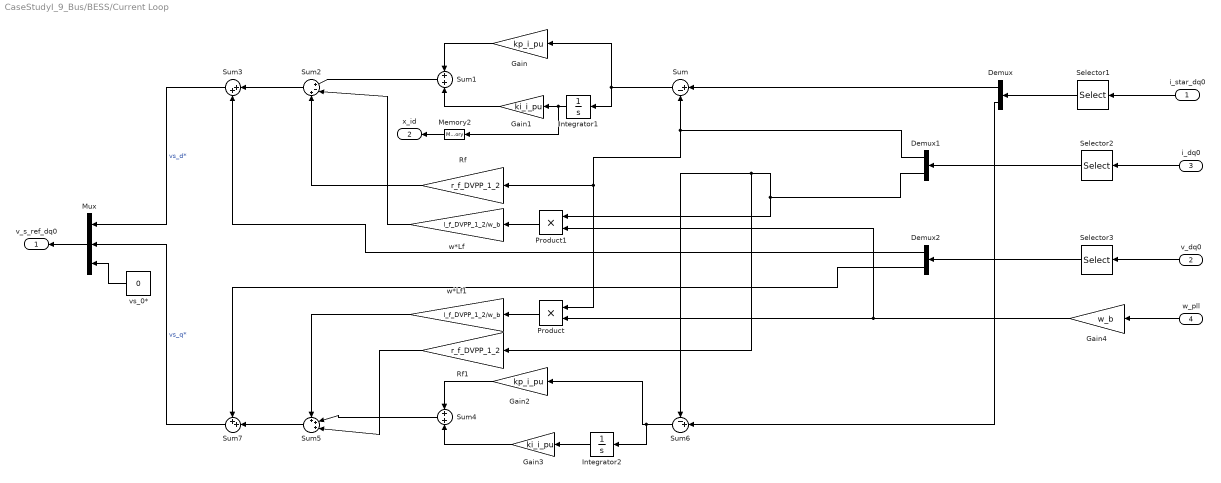
== system CaseStudyI_9_Bus/BESS/Current Loop ==
  i_star_dq0 : Inport
  v_dq0 : Inport  Port=2
  i_dq0 : Inport  Port=3
  w_pll : Inport  Port=4
  Demux : Demux  Outputs=2
  Demux1 : Demux  Outputs=2
  Demux2 : Demux  Outputs=2
  Gain : Gain  Gain=kp_i_pu
  Gain1 : Gain  Gain=ki_i_pu
  Gain2 : Gain  Gain=kp_i_pu
  Gain3 : Gain  Gain=ki_i_pu
  Gain4 : Gain  Gain=w_b
  Integrator1 : Integrator  InitialCondition=xid0_DVPP_1_2_pu
  Integrator2 : Integrator  InitialCondition=xiq0_DVPP_1_2_pu
  Memory2 : Memory
  Mux : Mux  Inputs=3
  Product : Product
  Product1 : Product
  Rf : Gain  Gain=r_f_DVPP_1_2
  Rf1 : Gain  Gain=r_f_DVPP_1_2
  Selector1 : Selector  InputPortWidth=3  IndexOptions=Index vector (dialog)  Indices=[1 2]  OutputSizes=1
  Selector2 : Selector  InputPortWidth=3  IndexOptions=Index vector (dialog)  Indices=[1 2]  OutputSizes=1
  Selector3 : Selector  InputPortWidth=3  IndexOptions=Index vector (dialog)  Indices=[1 2]  OutputSizes=1
  Sum : Sum  Inputs=|+-
  Sum1 : Sum
  Sum2 : Sum  Inputs=|+-+
  Sum3 : Sum  Inputs=|++
  Sum4 : Sum
  Sum5 : Sum  Inputs=+++|
  Sum6 : Sum  Inputs=-+|
  Sum7 : Sum  Inputs=++|
  vs_0* : Constant  Value=0
  w*Lf : Gain  Gain=l_f_DVPP_1_2/w_b
  w*Lf1 : Gain  Gain=l_f_DVPP_1_2/w_b
  v_s_ref_dq0 : Outport  VectorParamsAs1DForOutWhenUnconnected=off
  x_id : Outport  Port=2  VectorParamsAs1DForOutWhenUnconnected=off
  wires:
  vs_0*/1 -> Mux/3
  Selector3/1 -> Demux2/1
  i_dq0/1 -> Selector2/1
  Selector2/1 -> Demux1/1
  Mux/1 -> v_s_ref_dq0/1
  Sum2/1 -> Sum3/1
  v_dq0/1 -> Selector3/1
  i_star_dq0/1 -> Selector1/1
  w*Lf/1 -> Sum2/2
  Sum7/1 -> Mux/2  "vs_q*"
  Sum3/1 -> Mux/1  "vs_d*"
  Sum5/1 -> Sum7/2
  Rf/1 -> Sum2/3
  Rf1/1 -> Sum5/3
  Sum/1 -> Integrator1/1, Gain/1
  Sum1/1 -> Sum2/1
  Selector1/1 -> Demux/1
  Demux/2 -> Sum6/2
  Demux/1 -> Sum/1
  w*Lf1/1 -> Sum5/1
  Demux2/1 -> Sum3/2
  Demux2/2 -> Sum7/1
  Demux1/1 -> Product/1, Rf/1, Sum/2
  Demux1/2 -> Product1/1, Rf1/1, Sum6/1
  Gain/1 -> Sum1/1
  Gain1/1 -> Sum1/2
  Gain2/1 -> Sum4/1
  Sum6/1 -> Integrator2/1, Gain2/1
  Sum4/1 -> Sum5/2
  Gain3/1 -> Sum4/2
  Integrator2/1 -> Gain3/1
  Integrator1/1 -> Memory2/1, Gain1/1
  w_pll/1 -> Gain4/1
  Product/1 -> w*Lf1/1
  Product1/1 -> w*Lf/1
  Gain4/1 -> Product1/2, Product/2
  Memory2/1 -> x_id/1

== system CaseStudyI_9_Bus/BESS/PLL ==
  v_abc : Inport
  Display : Display
  Gain : Gain  Gain=1/fb
  Integrator3 : Integrator  InitialCondition=xpll0_pu
  Selector : Selector  InputPortWidth=3  IndexOptions=Index vector (dialog)  Indices=2  OutputSizes=1
  Subsystem : Subsystem
  abc to dq0 : powerlib_meascontrol/Transformations/abc to dq0  Alignment=90 degrees behind phase A axis
  theta_pll : Outport  VectorParamsAs1DForOutWhenUnconnected=off
  v_dq0 : Outport  Port=2  VectorParamsAs1DForOutWhenUnconnected=off
  w_pll : Outport  Port=3  VectorParamsAs1DForOutWhenUnconnected=off
  x_pll : Outport  Port=4  VectorParamsAs1DForOutWhenUnconnected=off
  wires:
  Gain/1 -> w_pll/1
  Integrator3/1 -> x_pll/1
  v_abc/1 -> Subsystem/1(Vabc), abc to dq0/1
  abc to dq0/1 -> Selector/1, v_dq0/1
  Subsystem/1(Freq) -> Display/1, Gain/1
  Subsystem/2(wt) -> abc to dq0/2, theta_pll/1
  Selector/1 -> Integrator3/1

== system CaseStudyI_9_Bus/BESS/Power Controllers ==
  Q_abc : Inport
  P_abc : Inport  Port=2
  Q_set : Inport  Port=3
  Delta x_c : Inport  Port=4
  w_pll : Inport  Port=5
  P_set : Inport  Port=6
  0 : Constant  Value=0
  DVPP State Feedback Controller for Active Power Control : Subsystem
  Mux : Mux  Inputs=3
  Reactive Power Controller PI-droop control : Subsystem
  i_star_dq0 : Outport
  p_des : Outport  Port=2
  wires:
  Mux/1 -> i_star_dq0/1
  0/1 -> Mux/3
  DVPP State Feedback Controller for Active Power Control/1(p_des) -> p_des/1
  w_pll/1 -> DVPP State Feedback Controller for Active Power Control/3(w_pll)
  P_abc/1 -> DVPP State Feedback Controller for Active Power Control/1(P_abc)
  Reactive Power Controller PI-droop control/1(i_star_q) -> Mux/2
  Q_abc/1 -> Reactive Power Controller PI-droop control/1(Q_abc)
  Q_set/1 -> Reactive Power Controller PI-droop control/2(Qset)
  Delta x_c/1 -> DVPP State Feedback Controller for Active Power Control/2(Delta_x_c)
  DVPP State Feedback Controller for Active Power Control/2(i_star_d) -> Mux/1
  P_set/1 -> DVPP State Feedback Controller for Active Power Control/4(Pset)

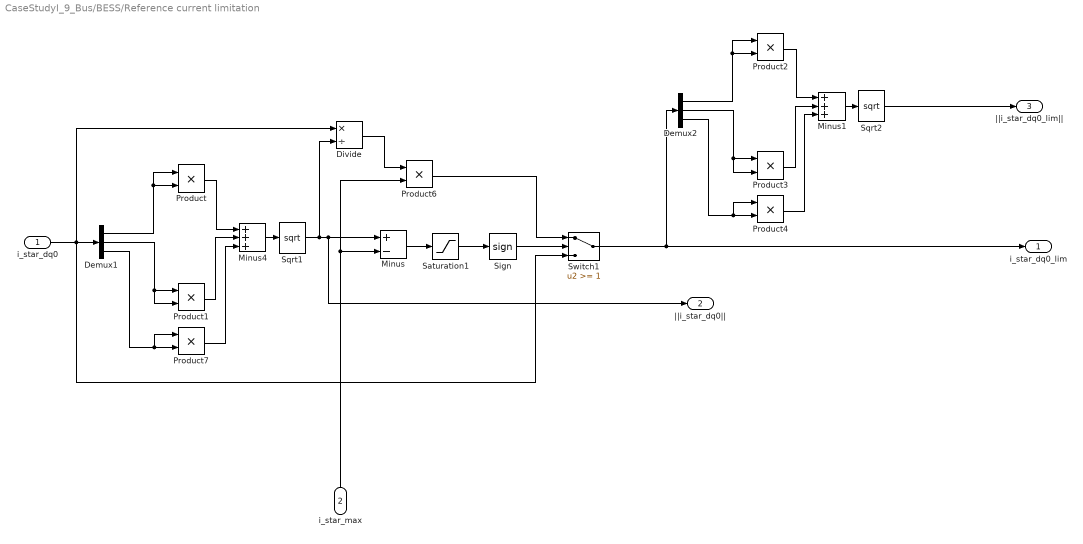
== system CaseStudyI_9_Bus/BESS/Reference current limitation ==
  i_star_dq0 : Inport
  i_star_max : Inport  Port=2
  Demux1 : Demux  Outputs=3
  Demux2 : Demux  Outputs=3
  Divide : Product  Inputs=*/
  Minus : Sum  Inputs=+-
  Minus1 : Sum  Inputs=+++
  Minus4 : Sum  Inputs=+++
  Product{,1..4,6..7} (7 alike) : Product  RndMeth=Zero
  Saturation1 : Saturate  UpperLimit=inf  LowerLimit=0
  Sign : Signum
  Sqrt1 : Sqrt  SaturateOnIntegerOverflow=on
  Sqrt2 : Sqrt  SaturateOnIntegerOverflow=on
  Switch1 : Switch  Threshold=1
  i_star_dq0_lim : Outport  VectorParamsAs1DForOutWhenUnconnected=off
  ||i_star_dq0|| : Outport  Port=2  VectorParamsAs1DForOutWhenUnconnected=off
  ||i_star_dq0_lim|| : Outport  Port=3  VectorParamsAs1DForOutWhenUnconnected=off
  wires:
  Sqrt2/1 -> ||i_star_dq0_lim||/1
  Minus1/1 -> Sqrt2/1
  Demux2/2 -> Product3/2, Product3/1
  Product3/1 -> Minus1/2
  Demux2/1 -> Product2/1, Product2/2
  Product4/1 -> Minus1/3
  Demux2/3 -> Product4/2, Product4/1
  Product2/1 -> Minus1/1
  i_star_max/1 -> Product6/2, Minus/2
  i_star_dq0/1 -> Switch1/3, Demux1/1, Divide/1
  Switch1/1 -> i_star_dq0_lim/1, Demux2/1
  Demux1/3 -> Product7/2, Product7/1
  Product7/1 -> Minus4/3
  Product6/1 -> Switch1/1
  Divide/1 -> Product6/1
  Sign/1 -> Switch1/2
  Saturation1/1 -> Sign/1
  Demux1/2 -> Product1/2, Product1/1
  Product/1 -> Minus4/1
  Product1/1 -> Minus4/2
  Demux1/1 -> Product/1, Product/2
  Minus4/1 -> Sqrt1/1
  Sqrt1/1 -> Minus/1, ||i_star_dq0||/1, Divide/2
  Minus/1 -> Saturation1/1

== system CaseStudyI_9_Bus/Supercapacitor/Converter State Deviation ==
  i_dq0 : Inport
  x_id : Inport  Port=2
  pset : Inport  Port=3
  Constant1 : Constant  Value=xid0_DVPP_1_3_pu
  Demux2 : Demux  Outputs=3
  Gain : Gain  Gain=1/vd0_DVPP_1_3_pu
  Mux : Mux  Inputs=2
  Sum : Sum  Inputs=-+|
  Sum1 : Sum  Inputs=|+-
  Delta x_c : Outport
  wires:
  i_dq0/1 -> Demux2/1
  pset/1 -> Gain/1
  Sum/1 -> Mux/1
  Demux2/1 -> Sum/2
  Gain/1 -> Sum/1
  x_id/1 -> Sum1/1
  Constant1/1 -> Sum1/2
  Mux/1 -> Delta x_c/1
  Sum1/1 -> Mux/2

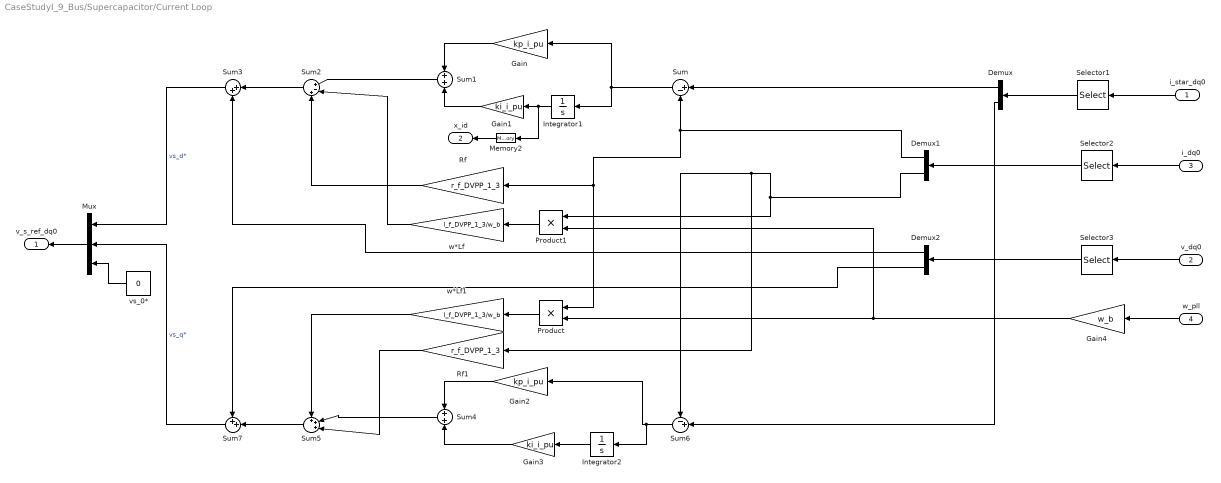
== system CaseStudyI_9_Bus/Supercapacitor/Current Loop ==
  i_star_dq0 : Inport
  v_dq0 : Inport  Port=2
  i_dq0 : Inport  Port=3
  w_pll : Inport  Port=4
  Demux : Demux  Outputs=2
  Demux1 : Demux  Outputs=2
  Demux2 : Demux  Outputs=2
  Gain : Gain  Gain=kp_i_pu
  Gain1 : Gain  Gain=ki_i_pu
  Gain2 : Gain  Gain=kp_i_pu
  Gain3 : Gain  Gain=ki_i_pu
  Gain4 : Gain  Gain=w_b
  Integrator1 : Integrator  InitialCondition=xid0_DVPP_1_3_pu
  Integrator2 : Integrator  InitialCondition=xiq0_DVPP_1_3_pu
  Memory2 : Memory
  Mux : Mux  Inputs=3
  Product : Product
  Product1 : Product
  Rf : Gain  Gain=r_f_DVPP_1_3
  Rf1 : Gain  Gain=r_f_DVPP_1_3
  Selector1 : Selector  InputPortWidth=3  IndexOptions=Index vector (dialog)  Indices=[1 2]  OutputSizes=1
  Selector2 : Selector  InputPortWidth=3  IndexOptions=Index vector (dialog)  Indices=[1 2]  OutputSizes=1
  Selector3 : Selector  InputPortWidth=3  IndexOptions=Index vector (dialog)  Indices=[1 2]  OutputSizes=1
  Sum : Sum  Inputs=|+-
  Sum1 : Sum
  Sum2 : Sum  Inputs=|+-+
  Sum3 : Sum  Inputs=|++
  Sum4 : Sum
  Sum5 : Sum  Inputs=+++|
  Sum6 : Sum  Inputs=-+|
  Sum7 : Sum  Inputs=++|
  vs_0* : Constant  Value=0
  w*Lf : Gain  Gain=l_f_DVPP_1_3/w_b
  w*Lf1 : Gain  Gain=l_f_DVPP_1_3/w_b
  v_s_ref_dq0 : Outport  VectorParamsAs1DForOutWhenUnconnected=off
  x_id : Outport  Port=2  VectorParamsAs1DForOutWhenUnconnected=off
  wires:
  vs_0*/1 -> Mux/3
  Selector3/1 -> Demux2/1
  i_dq0/1 -> Selector2/1
  Selector2/1 -> Demux1/1
  Mux/1 -> v_s_ref_dq0/1
  Sum2/1 -> Sum3/1
  v_dq0/1 -> Selector3/1
  i_star_dq0/1 -> Selector1/1
  w*Lf/1 -> Sum2/2
  Sum7/1 -> Mux/2  "vs_q*"
  Sum3/1 -> Mux/1  "vs_d*"
  Sum5/1 -> Sum7/2
  Rf/1 -> Sum2/3
  Rf1/1 -> Sum5/3
  Sum/1 -> Integrator1/1, Gain/1
  Sum1/1 -> Sum2/1
  Selector1/1 -> Demux/1
  Demux/2 -> Sum6/2
  Demux/1 -> Sum/1
  w*Lf1/1 -> Sum5/1
  Demux2/1 -> Sum3/2
  Demux2/2 -> Sum7/1
  Demux1/1 -> Product/1, Rf/1, Sum/2
  Demux1/2 -> Product1/1, Rf1/1, Sum6/1
  Gain/1 -> Sum1/1
  Gain1/1 -> Sum1/2
  Gain2/1 -> Sum4/1
  Sum6/1 -> Integrator2/1, Gain2/1
  Sum4/1 -> Sum5/2
  Gain3/1 -> Sum4/2
  Integrator2/1 -> Gain3/1
  Integrator1/1 -> Memory2/1, Gain1/1
  w_pll/1 -> Gain4/1
  Product/1 -> w*Lf1/1
  Product1/1 -> w*Lf/1
  Gain4/1 -> Product1/2, Product/2
  Memory2/1 -> x_id/1

== system CaseStudyI_9_Bus/Supercapacitor/PLL ==
  v_abc : Inport
  Display : Display
  Gain : Gain  Gain=1/fb
  Integrator3 : Integrator  InitialCondition=xpll0_pu
  Selector : Selector  InputPortWidth=3  IndexOptions=Index vector (dialog)  Indices=2  OutputSizes=1
  Subsystem : Subsystem
  abc to dq0 : powerlib_meascontrol/Transformations/abc to dq0  Alignment=90 degrees behind phase A axis
  theta_pll : Outport  VectorParamsAs1DForOutWhenUnconnected=off
  v_dq0 : Outport  Port=2  VectorParamsAs1DForOutWhenUnconnected=off
  w_pll : Outport  Port=3  VectorParamsAs1DForOutWhenUnconnected=off
  x_pll : Outport  Port=4  VectorParamsAs1DForOutWhenUnconnected=off
  wires:
  Gain/1 -> w_pll/1
  Integrator3/1 -> x_pll/1
  v_abc/1 -> Subsystem/1(Vabc), abc to dq0/1
  abc to dq0/1 -> Selector/1, v_dq0/1
  Subsystem/1(Freq) -> Display/1, Gain/1
  Subsystem/2(wt) -> abc to dq0/2, theta_pll/1
  Selector/1 -> Integrator3/1

== system CaseStudyI_9_Bus/Supercapacitor/Power Controllers ==
  Q_abc : Inport
  w_pll : Inport  Port=2
  P_abc : Inport  Port=3
  Q_set : Inport  Port=4
  Delta x_c : Inport  Port=5
  P_set : Inport  Port=6
  0 : Constant  Value=0
  DVPP State Feedback Controller for Active Power Control : Subsystem
  Mux : Mux  Inputs=3
  Reactive Power Controller PI-droop control : Subsystem
  i_star_dq0 : Outport
  p_des : Outport  Port=2
  wires:
  Mux/1 -> i_star_dq0/1
  0/1 -> Mux/3
  DVPP State Feedback Controller for Active Power Control/2(i_star_d) -> Mux/1
  DVPP State Feedback Controller for Active Power Control/1(p_des) -> p_des/1
  w_pll/1 -> DVPP State Feedback Controller for Active Power Control/1(w_pll)
  P_abc/1 -> DVPP State Feedback Controller for Active Power Control/2(P_abc)
  Reactive Power Controller PI-droop control/1(i_star_q) -> Mux/2
  Q_abc/1 -> Reactive Power Controller PI-droop control/1(Q_abc)
  Q_set/1 -> Reactive Power Controller PI-droop control/2(Qset)
  Delta x_c/1 -> DVPP State Feedback Controller for Active Power Control/3(Delta_x_c)
  P_set/1 -> DVPP State Feedback Controller for Active Power Control/4(P_set)

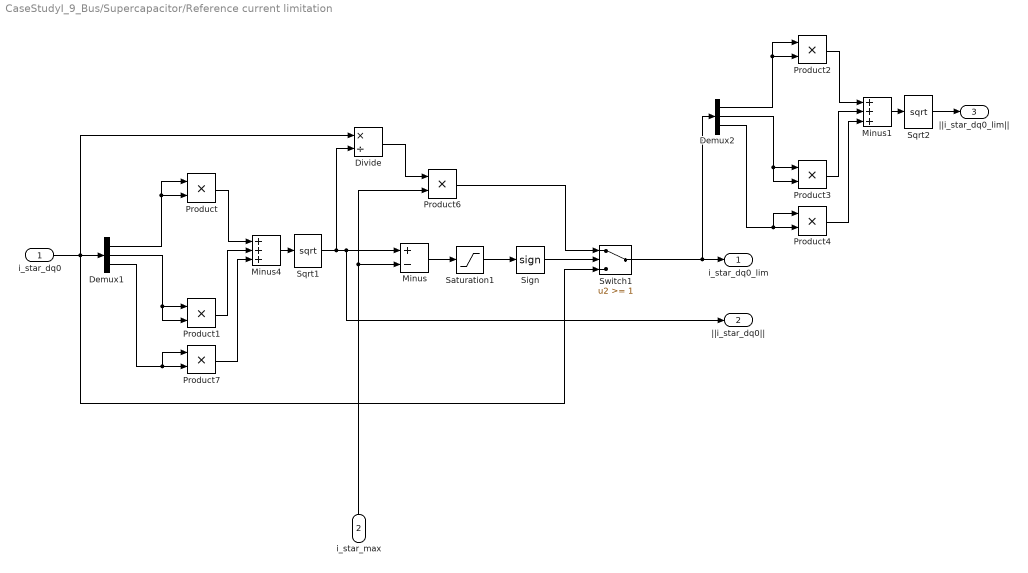
== system CaseStudyI_9_Bus/Supercapacitor/Reference current limitation ==
  i_star_dq0 : Inport
  i_star_max : Inport  Port=2
  Demux1 : Demux  Outputs=3
  Demux2 : Demux  Outputs=3
  Divide : Product  Inputs=*/
  Minus : Sum  Inputs=+-
  Minus1 : Sum  Inputs=+++
  Minus4 : Sum  Inputs=+++
  Product{,1..4,6..7} (7 alike) : Product  RndMeth=Zero
  Saturation1 : Saturate  UpperLimit=inf  LowerLimit=0
  Sign : Signum
  Sqrt1 : Sqrt  SaturateOnIntegerOverflow=on
  Sqrt2 : Sqrt  SaturateOnIntegerOverflow=on
  Switch1 : Switch  Threshold=1
  i_star_dq0_lim : Outport  VectorParamsAs1DForOutWhenUnconnected=off
  ||i_star_dq0|| : Outport  Port=2  VectorParamsAs1DForOutWhenUnconnected=off
  ||i_star_dq0_lim|| : Outport  Port=3  VectorParamsAs1DForOutWhenUnconnected=off
  wires:
  Sqrt2/1 -> ||i_star_dq0_lim||/1
  Minus1/1 -> Sqrt2/1
  Demux2/2 -> Product3/2, Product3/1
  Product3/1 -> Minus1/2
  Demux2/1 -> Product2/1, Product2/2
  Product4/1 -> Minus1/3
  Demux2/3 -> Product4/2, Product4/1
  Product2/1 -> Minus1/1
  i_star_max/1 -> Product6/2, Minus/2
  i_star_dq0/1 -> Switch1/3, Demux1/1, Divide/1
  Switch1/1 -> i_star_dq0_lim/1, Demux2/1
  Demux1/3 -> Product7/2, Product7/1
  Product7/1 -> Minus4/3
  Product6/1 -> Switch1/1
  Divide/1 -> Product6/1
  Sign/1 -> Switch1/2
  Saturation1/1 -> Sign/1
  Demux1/2 -> Product1/2, Product1/1
  Product/1 -> Minus4/1
  Product1/1 -> Minus4/2
  Demux1/1 -> Product/1, Product/2
  Minus4/1 -> Sqrt1/1
  Sqrt1/1 -> Minus/1, ||i_star_dq0||/1, Divide/2
  Minus/1 -> Saturation1/1
